simulink model "LQG_P1_faster"  (R2019a)
settings: Solver=VariableStepAuto  StartTime=0.0  StopTime=10  RelTol=1e-3
settings Model: Creator=morga  LastModifiedBy=morga

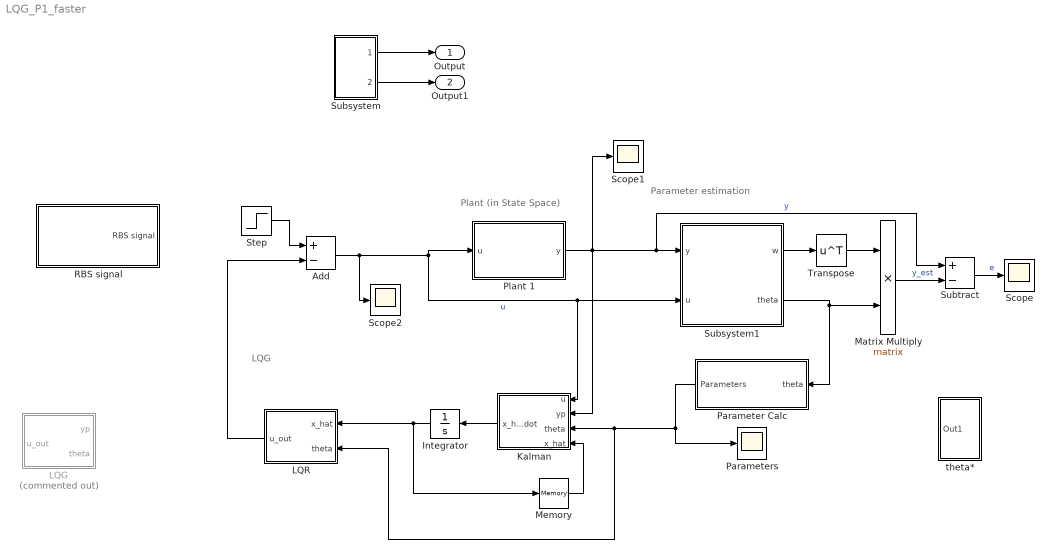
== system LQG_P1_faster ==
  note: LQG
  note: Parameter estimation
  note: Plant (in State Space)
  Add : Sum  Inputs=+-
  Integrator : Integrator
  Kalman : MATLAB Function  TreatAsAtomicUnit=on
  LQG : MATLAB Function  Commented=on  TreatAsAtomicUnit=on
  LQR : MATLAB Function  TreatAsAtomicUnit=on
  Matrix Multiply : Product  Multiplication=Matrix(*)
  Memory : Memory  InitialCondition=[0 0]'
  Parameter Calc : Subsystem
  Parameters : Scope
  Plant 1 : Subsystem
  RBS signal : Subsystem
  Scope : Scope
  Scope1 : Scope
  Scope2 : Scope
  Step : Step  Time=0  SampleTime=0
  Subsystem : Subsystem
  Subsystem1 : Subsystem
  Subtract : Sum  Inputs=+-
  Transpose : Math  Operator=transpose  SaturateOnIntegerOverflow=on
  theta* : Subsystem
  Output : Outport
  Output1 : Outport  Port=2
  wires:
  Plant 1/1(y) -> Scope1/1, Kalman/2(yp), Subtract/1, Subsystem1/1(y)  "y"
  Add/1 -> Scope2/1, Plant 1/1(u), Kalman/1(u), Subsystem1/2(u)  "u"
  Subtract/1 -> Scope/1  "e"
  Step/1 -> Add/1
  Parameter Calc/1(Parameters) -> Kalman/3(theta), LQR/2(theta), Parameters/1
  Subsystem/2(Output1) -> Output1/1
  Transpose/1 -> Matrix Multiply/1
  Subsystem1/2(theta) -> Parameter Calc/1(theta), Matrix Multiply/2
  Matrix Multiply/1 -> Subtract/2  "y_est"
  Subsystem1/1(w) -> Transpose/1
  Subsystem/1(Output) -> Output/1
  LQR/1(u_out) -> Add/2
  Memory/1 -> Kalman/4(x_hat)
  Kalman/1(x_hat_dot) -> Integrator/1
  Integrator/1 -> LQR/1(x_hat), Memory/1

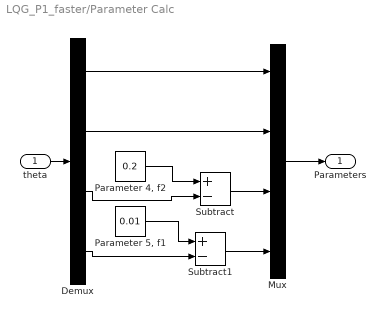
== system LQG_P1_faster/Parameter Calc ==
  theta : Inport
  Demux : Demux
  Mux : Mux
  "Parameter 4, f2" : Constant  Value=0.2
  "Parameter 5, f1" : Constant  Value=0.01
  Subtract : Sum  Inputs=+-
  Subtract1 : Sum  Inputs=+-
  Parameters : Outport
  wires:
  theta/1 -> Demux/1
  Demux/1 -> Mux/1
  Demux/2 -> Mux/2
  "Parameter 4, f2"/1 -> Subtract/1
  "Parameter 5, f1"/1 -> Subtract1/1
  Demux/4 -> Subtract1/2
  Demux/3 -> Subtract/2
  Subtract/1 -> Mux/3
  Subtract1/1 -> Mux/4
  Mux/1 -> Parameters/1

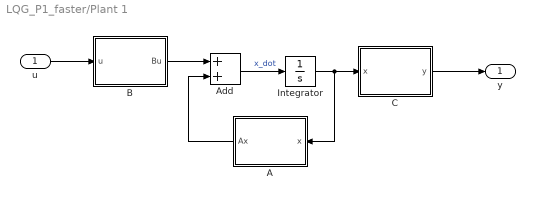
== system LQG_P1_faster/Plant 1 ==
  u : Inport  PortDimensions=1
  A : MATLAB Function  TreatAsAtomicUnit=on
  Add : Sum
  B : MATLAB Function  TreatAsAtomicUnit=on
  C : MATLAB Function  TreatAsAtomicUnit=on
  Integrator : Integrator  InitialCondition=[0 0]
  y : Outport
  wires:
  B/1(Bu) -> Add/1
  A/1(Ax) -> Add/2
  Add/1 -> Integrator/1  "x_dot"
  Integrator/1 -> A/1(x), C/1(x)
  C/1(y) -> y/1
  u/1 -> B/1(u)

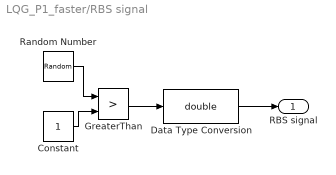
== system LQG_P1_faster/RBS signal ==
  Constant : Constant
  Data Type Conversion : DataTypeConversion  OutDataTypeStr=double
  GreaterThan : RelationalOperator  Operator=>  OutDataTypeStr=boolean  RndMeth=Simplest
  Random Number : RandomNumber  Mean=1  SampleTime=0.1
  RBS signal : Outport
  wires:
  Random Number/1 -> GreaterThan/1
  Data Type Conversion/1 -> RBS signal/1
  GreaterThan/1 -> Data Type Conversion/1
  Constant/1 -> GreaterThan/2

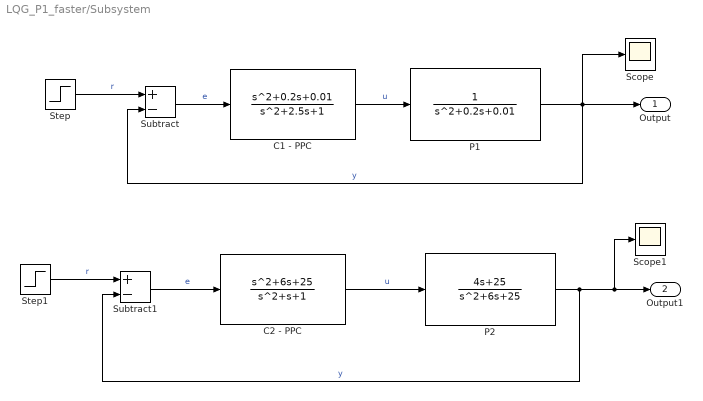
== system LQG_P1_faster/Subsystem ==
  C1 - PPC : TransferFcn  Numerator=[1 0.2 0.01]  Denominator=[1 2.5 1]
  C2 - PPC : TransferFcn  Numerator=[1 6 25]  Denominator=[1 1 1]
  P1 : TransferFcn  Denominator=[1 0.2 0.01]
  P2 : TransferFcn  Numerator=[4 25]  Denominator=[1 6 25]
  Scope : Scope
  Scope1 : Scope
  Step : Step  SampleTime=0
  Step1 : Step  SampleTime=0
  Subtract : Sum  Inputs=+-
  Subtract1 : Sum  Inputs=+-
  Output : Outport
  Output1 : Outport  Port=2
  wires:
  C1 - PPC/1 -> P1/1  "u"
  P1/1 -> Output/1, Scope/1, Subtract/2  "y"
  P2/1 -> Output1/1, Scope1/1, Subtract1/2  "y"
  Step/1 -> Subtract/1  "r"
  C2 - PPC/1 -> P2/1  "u"
  Subtract/1 -> C1 - PPC/1  "e"
  Subtract1/1 -> C2 - PPC/1  "e"
  Step1/1 -> Subtract1/1  "r"

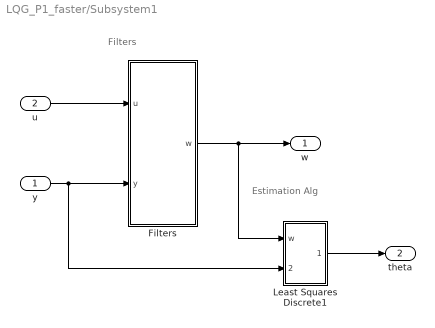
== system LQG_P1_faster/Subsystem1 ==
  note: Estimation Alg
  note: Filters
  y : Inport
  u : Inport  Port=2
  Filters : Subsystem
  Least Squares Discrete1 : Subsystem
  w : Outport
  theta : Outport  Port=2
  wires:
  u/1 -> Filters/1(u)
  y/1 -> Least Squares Discrete1/2(Y_p), Filters/2(y)
  Filters/1(w) -> w/1, Least Squares Discrete1/1(w)
  Least Squares Discrete1/1(theta) -> theta/1

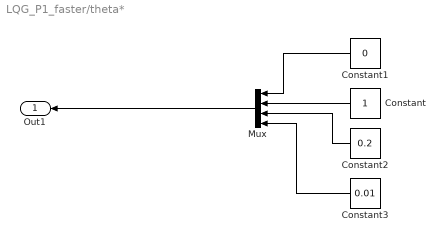
== system LQG_P1_faster/theta* ==
  Constant : Constant
  Constant1 : Constant  Value=0
  Constant2 : Constant  Value=0.2
  Constant3 : Constant  Value=0.01
  Mux : Mux
  Out1 : Outport
  wires:
  Constant/1 -> Mux/2
  Constant3/1 -> Mux/4
  Constant2/1 -> Mux/3
  Constant1/1 -> Mux/1
  Mux/1 -> Out1/1

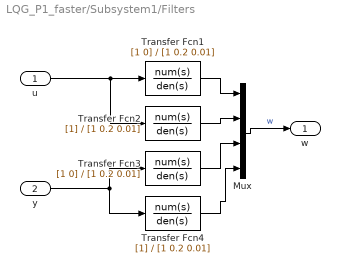
== system LQG_P1_faster/Subsystem1/Filters ==
  u : Inport  PortDimensions=1
  y : Inport  Port=2
  Mux : Mux
  Transfer Fcn1 : TransferFcn  Numerator=[1 0]  Denominator=[1 0.2 0.01]
  Transfer Fcn2 : TransferFcn  Denominator=[1 0.2 0.01]
  Transfer Fcn3 : TransferFcn  Numerator=[1 0]  Denominator=[1 0.2 0.01]
  Transfer Fcn4 : TransferFcn  Denominator=[1 0.2 0.01]
  w : Outport
  wires:
  Transfer Fcn2/1 -> Mux/2
  u/1 -> Transfer Fcn2/1, Transfer Fcn1/1
  Transfer Fcn3/1 -> Mux/3
  y/1 -> Transfer Fcn3/1, Transfer Fcn4/1
  Transfer Fcn1/1 -> Mux/1
  Mux/1 -> w/1  "w"
  Transfer Fcn4/1 -> Mux/4

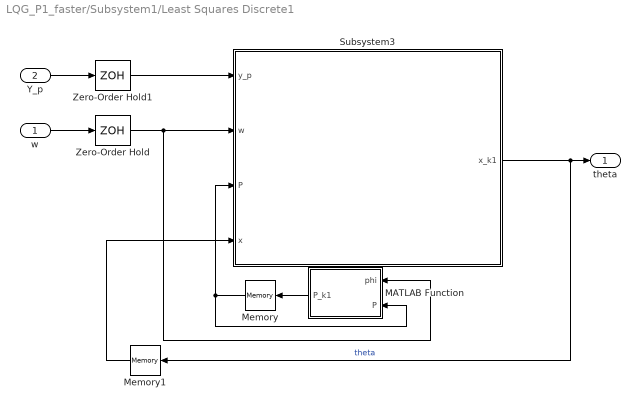
== system LQG_P1_faster/Subsystem1/Least Squares Discrete1 ==
  w : Inport
  Y_p : Inport  Port=2
  MATLAB Function : MATLAB Function  TreatAsAtomicUnit=on
  Memory : Memory  InitialCondition=100000*eye(4)
  Memory1 : Memory  InitialCondition=[0 0 0 0]
  Subsystem3 : Subsystem
  Zero-Order Hold : ZeroOrderHold  SampleTime=0.01
  Zero-Order Hold1 : ZeroOrderHold  SampleTime=0.01
  theta : Outport
  wires:
  Subsystem3/1(x_k1) -> Memory1/1, theta/1  "theta"
  MATLAB Function/1(P_k1) -> Memory/1
  w/1 -> Zero-Order Hold/1
  Zero-Order Hold1/1 -> Subsystem3/1(y_p)
  Memory/1 -> Subsystem3/3(P), MATLAB Function/2(P)
  Zero-Order Hold/1 -> MATLAB Function/1(phi), Subsystem3/2(w)
  Y_p/1 -> Zero-Order Hold1/1
  Memory1/1 -> Subsystem3/4(x)

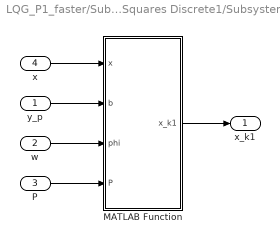
== system LQG_P1_faster/Subsystem1/Least Squares Discrete1/Subsystem3 ==
  y_p : Inport
  w : Inport  Port=2
  P : Inport  Port=3
  x : Inport  Port=4
  MATLAB Function : MATLAB Function  TreatAsAtomicUnit=on
  x_k1 : Outport
  wires:
  MATLAB Function/1(x_k1) -> x_k1/1
  y_p/1 -> MATLAB Function/2(b)
  P/1 -> MATLAB Function/4(P)
  w/1 -> MATLAB Function/3(phi)
  x/1 -> MATLAB Function/1(x)

== matlab function LQG_P1_faster/Subsystem1/Least Squares Discrete1/MATLAB Function ==
  data: phi input; P_k1 output; P input
function P_k1 = fcn(phi,P)
alpha = 1;
lambda = 1;

P_k1 = 1/alpha*P - (lambda*lambda*P*phi*phi'*P)/(1+lambda*phi'*P*phi);

== matlab function LQG_P1_faster/LQR ==
  data: x_hat input; theta input; u_out output
function u_out = fcn(x_hat, theta)
coder.extrinsic('lqr');
u_out = 0;

A = [0 1; -theta(4) -theta(3)];
B = [0; 1];
Q = eye(2);
R = [1];
K = lqr(A,B,Q,R); %LQR controller gain

u_out = K * x_hat;
end

== matlab function LQG_P1_faster/Plant 1/A ==
  data: x input; Ax output
function Ax = fcn(x)
A = [0 1; -0.01 -0.2];
Ax = A*x;

== matlab function LQG_P1_faster/Plant 1/B ==
  data: u input; Bu output
function Bu = fcn(u)
B = [0 1]';
Bu = B*u;

== matlab function LQG_P1_faster/Plant 1/C ==
  data: x input; y output
function y = fcn(x)
C = [1 0];
y = C*x;

== matlab function LQG_P1_faster/Kalman ==
  data: u input; yp input; theta input; x_hat_dot output; x_hat input
function x_hat_dot = fcn(u, yp, theta, x_hat)
coder.extrinsic('kalman', 'ss');
x_hat_dot = [0 0]';
L = [0 0]';

% This part is for the Kalman filter for state estimation
A = [0 1; -theta(4) -theta(3)];
B = [0; 1];
C = [theta(2) theta(1)];
sys = ss(A, B, C, 0);
Qn = 1; Rn = [0.01]; %noise covariance matrices for Kalman filter
[kest, L, P] = kalman(sys, Qn, Rn);

x_hat_dot = A*x_hat + B*u + L*(yp - C*x_hat);
end

== matlab function LQG_P1_faster/Subsystem1/Least Squares Discrete1/Subsystem3/MATLAB Function ==
  data: x input; x_k1 output; b input; phi input; P input
function x_k1 = fcn(x,b,phi,P)
lambda = 1; 
% X_k1 = theta_k+1
% b = y(t)

x_k1 = x - (lambda*P*phi*(phi'*x-b))/(1+lambda*phi'*P*phi);

== matlab function LQG_P1_faster/LQG ==
  data: yp input; theta input; u_out output
function u_out = fcn(yp, theta)
coder.extrinsic('lqr', 'kalman', 'ss');
u_out = 0;
% u_output = (LQG_control(theta, yp));

B = [0; 1];
a0 = theta(4); a1 = theta(3); %values of A in CCF 
A = [0 1; -a0 -a1];
Q = eye(2);
R = [1];
K = lqr(A,B,Q,R); %LQR controller gain

% This part is for the Kalman filter for state estimation
C = [theta(2) theta(1)];
sys = ss(A, B, C, 0);
Qn = 1; Rn = [0.01];
[kest, L, P] = kalman(sys, Qn, Rn);
L = L * -1;
K = K*-1;

%regulator = lqgreg(kest, K); %forms LQG regulator controller/estimator

x_hat = L * yp;
u_out = K * x_hat;
end
